simulink model "HW7_F_f_d"  (R2018a)
settings: Solver=VariableStepAuto  StartTime=0.0  StopTime=100  RelTol=1e-3
InitFcn:
  | vtol_param
  | F_f
  | F_f_b
StartFcn:
  | vtol_param
  | F_f
  | F_f_b
undefined symbols (not defined in the file or in its folder): Kh, Kth, Kz, P, phlead, PlotVtol, pth, pz, zhlead, zth, zz
ContinueFcn:
  | FT2frfl
settings Model: Creator=sadam  LastModifiedBy=sadam

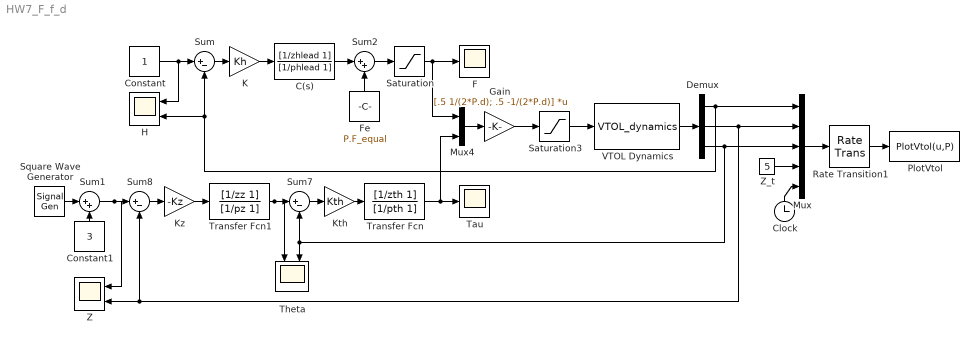
== system HW7_F_f_d ==
  C(s) : TransferFcn  Numerator=[1/zhlead 1]  Denominator=[1/phlead 1]
  Clock : Clock
  Constant : Constant
  Constant1 : Constant  Value=3
  Demux : Demux  Outputs=3
  F : Scope
  Fe : Constant  Value=P.F_equal
  Gain : Gain  Gain=[.5 1/(2*P.d); .5 -1/(2*P.d)]  Multiplication=Matrix(K*u)
  "H " : Scope  NumInputPorts=2
  K : Gain  Gain=Kh
  Kth : Gain  Gain=Kth
  Kz : Gain  Gain=-Kz
  Mux : Mux  Inputs=5
  Mux4 : Mux  Inputs=2
  "PlotVtol " : MATLABFcn  MATLABFcn=PlotVtol(u,P)  OutputDimensions=0
  Rate Transition1 : RateTransition  OutPortSampleTime=P.t_plot
  Saturation : Saturate  UpperLimit=P.Force_max  LowerLimit=-P.Force_max
  Saturation3 : Saturate  UpperLimit=P.Force_max  LowerLimit=-P.Force_max
  Square Wave Generator : SignalGenerator  WaveForm=square  Amplitude=2  Frequency=.15/2
  Sum : Sum  Inputs=|+-
  Sum1 : Sum  Inputs=|++
  Sum2 : Sum  Inputs=|++
  Sum7 : Sum  Inputs=|+-
  Sum8 : Sum  Inputs=|+-
  Tau : Scope
  "Theta " : Scope  NumInputPorts=2
  Transfer Fcn : TransferFcn  Numerator=[1/zth 1]  Denominator=[1/pth 1]
  Transfer Fcn1 : TransferFcn  Numerator=[1/zz 1]  Denominator=[1/pz 1]
  VTOL Dynamics : S-Function  FunctionName=VTOL_dynamics  Parameters=P  SFunctionDeploymentMode=off  EnableBusSupport=off
  Z : Scope  NumInputPorts=2
  Z_t : Constant  Value=5
  wires:
  Mux/1 -> Rate Transition1/1
  VTOL Dynamics/1 -> Demux/1
  Rate Transition1/1 -> "PlotVtol "/1
  Z_t/1 -> Mux/4
  Clock/1 -> Mux/5
  Demux/1 -> Mux/1, Sum/2, "H "/2
  Demux/2 -> Mux/2, Z/2, Sum8/2
  Demux/3 -> Mux/3, "Theta "/2, Sum7/2
  Saturation3/1 -> VTOL Dynamics/1
  Gain/1 -> Saturation3/1
  Mux4/1 -> Gain/1
  Kth/1 -> Transfer Fcn/1
  Kz/1 -> Transfer Fcn1/1
  Sum7/1 -> Kth/1
  Transfer Fcn/1 -> Tau/1, Mux4/2
  Sum8/1 -> Kz/1
  Transfer Fcn1/1 -> "Theta "/1, Sum7/1
  Sum2/1 -> Saturation/1
  C(s)/1 -> Sum2/1
  Sum/1 -> K/1
  Fe/1 -> Sum2/2
  K/1 -> C(s)/1
  Constant/1 -> "H "/1, Sum/1
  Saturation/1 -> F/1, Mux4/1
  Sum1/1 -> Z/1, Sum8/1
  Square Wave Generator/1 -> Sum1/1
  Constant1/1 -> Sum1/2
